simulink model "duGimbal_read_Sensor_with_Due"  (R2024b)
settings: Solver=FixedStepDiscrete  StartTime=0.0  StopTime=Inf  FixedStep=1/1000  RelTol=1e-3
undefined symbols (not defined in the file): DiscIntNeverNeededParam
libraries: simulink_extras x4, Du_Gimbal_LIB x3, arduinolib x1
settings Model: ExtModeTrigDuration=2  Creator=leoni  LastModifiedBy=leoni
settings SolverCC: AutoInsertRateTranBlk=on
settings OptimizationCC: EnhancedBackFolding=on  PassReuseOutputArgsAs=Individual arguments  ZeroExternalMemoryAtStartup=off  ZeroInternalMemoryAtStartup=off  MaxStackSize=64  OptimizeBlockOrder=speed  DifferentSizesBufferReuse=on  OptimizationCustomize=off  EfficientTunableParamExpr=on
settings DebuggingCC: ParameterTunabilityLossMsg=error
settings HardwareCC: ProdBitPerPointer=32  ProdBitPerSizeT=32  ProdBitPerPtrDiffT=32  ProdLargestAtomicInteger=Long  ProdLargestAtomicFloat=Double  ProdWordSize=32  ProdHWDeviceType=ARM Compatible->ARM Cortex
settings SFSimCC: MATLABDynamicMemAlloc=off
settings RTWCC: Description=Embedded Coder  SystemTargetFile=ert.tlc  HardwareBoard=Arduino Due  TemplateMakefile=ert_default_tmf  Toolchain=Arduino ARM  BuildConfiguration=Faster Runs
settings CodeAppCC: ForceParamTrailComments=on  IgnoreCustomStorageClasses=off  OperatorAnnotations=on  SimulinkDataObjDesc=on  SFDataObjDesc=on  InsertBlockDesc=on
settings ERTTargetCC: SupportContinuousTime=on  SupportVariableSizeSignals=on  ExtModeTransport=3  ExtModeStaticAlloc=on  ExtModeAutomaticAllocSize=off  ExtModeStaticAllocSize=24576  ExtModeMexFile=ext_xcp  ExtModeIntrfLevel=Level2 - Open  InlinedParameterPlacement=Hierarchical

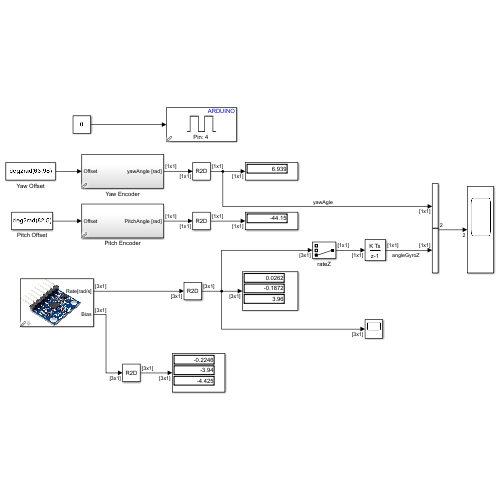
[thumbnail: Simulink's stored preview of the top-level diagram]
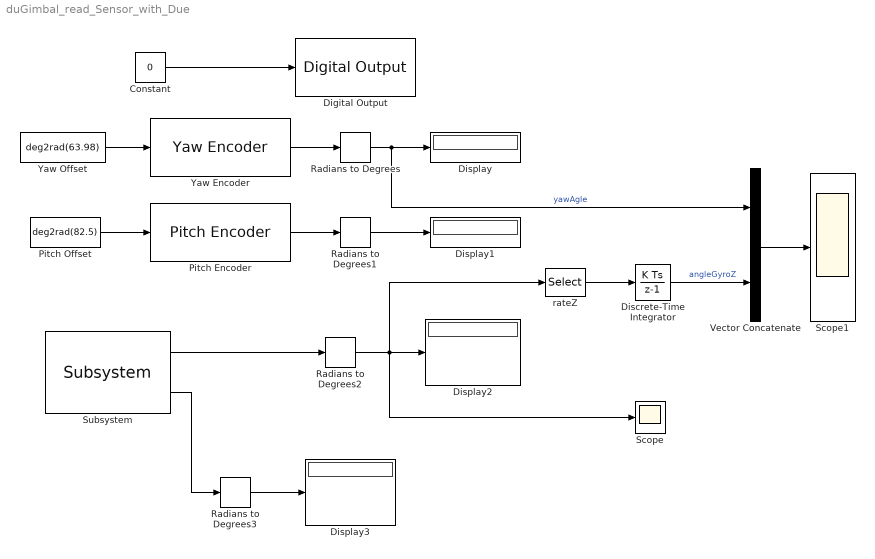
== system duGimbal_read_Sensor_with_Due ==
  Constant : Constant  Value=0
  Digital Output : arduinolib/Digital Output  pinNumber=4  Direction=output  blockPlatform=arduino
      settings: SourceProductName=Common
  Discrete-Time Integrator : DiscreteIntegrator  SampleTime=0.01  ICPrevOutput=DiscIntNeverNeededParam  ICPrevScaledInput=DiscIntNeverNeededParam
  Display{,1..3} (4 alike) : Display
  Pitch Encoder : Du_Gimbal_LIB/Pitch Encoder  SystemSampleTime=-1  VariantActivationTime=update diagram  AllowFlexibleInterface=on  Latency=0  AutoFrameSizeCalculation=off
  Pitch Offset : Constant  Value=deg2rad(82.5)
  Radians to Degrees{,1..3} (4 alike) : simulink_extras/Transformations/Radians to Degrees
  Scope : Scope
  Scope1 : Scope
  Subsystem : Du_Gimbal_LIB/Subsystem  ts=0.001  tInit=5
  Vector Concatenate : Concatenate
  Yaw Encoder : Du_Gimbal_LIB/Yaw Encoder  SystemSampleTime=-1  VariantActivationTime=update diagram  AllowFlexibleInterface=on  Latency=0  AutoFrameSizeCalculation=off
  Yaw Offset : Constant  Value=deg2rad(63.98)
  rateZ : Selector  InputPortWidth=3  IndexOptions=Index vector (dialog)  Indices=3  OutputSizes=1
  wires:
  Radians to Degrees/1 -> Vector Concatenate/1, Display/1  "yawAgle"
  Radians to Degrees1/1 -> Display1/1
  Yaw Encoder/1 -> Radians to Degrees/1
  Yaw Offset/1 -> Yaw Encoder/1
  Pitch Encoder/1 -> Radians to Degrees1/1
  Pitch Offset/1 -> Pitch Encoder/1
  Subsystem/1 -> Radians to Degrees2/1
  Radians to Degrees2/1 -> rateZ/1, Scope/1, Display2/1
  Subsystem/2 -> Radians to Degrees3/1
  Radians to Degrees3/1 -> Display3/1
  rateZ/1 -> Discrete-Time Integrator/1
  Discrete-Time Integrator/1 -> Vector Concatenate/2  "angleGyroZ"
  Vector Concatenate/1 -> Scope1/1
  Constant/1 -> Digital Output/1
